simulink model "Lecture_2_Exercises_Simulink"  (R2023b)
settings: Solver=ode3  StartTime=0.0  StopTime=100  FixedStep=0.001  RelTol=1e-3
values from neighbouring files (symbols this model uses):
  A = [ 0 1 ; -g/l*cos(pi/4) -d/(m*l^2) ]    [Lecture_2_Exercises.m]
  a = [m ... (first row only)    [Lecture_2_Exercises.m]
  B = [ 0 ; 1/(m*l^2) ]    [Lecture_2_Exercises.m]
  ustar = m*g*l*sin(xstar(1))    [Lecture_2_Exercises.m]
  xstar = [pi/4 ... (first row only)    [Lecture_2_Exercises.m]
libraries: simulink_extras x4
settings Model: Creator=therk  LastModifiedBy=therk

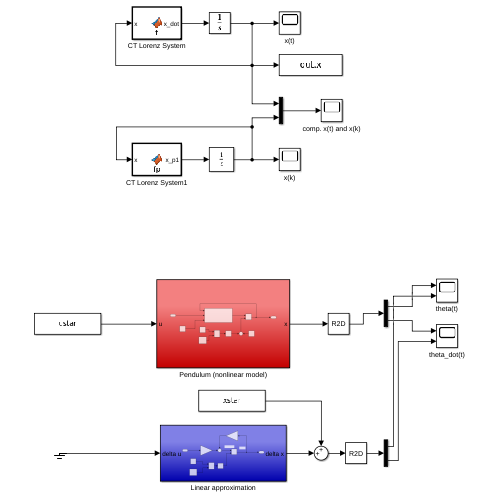
[thumbnail: Simulink's stored preview of the top-level diagram]
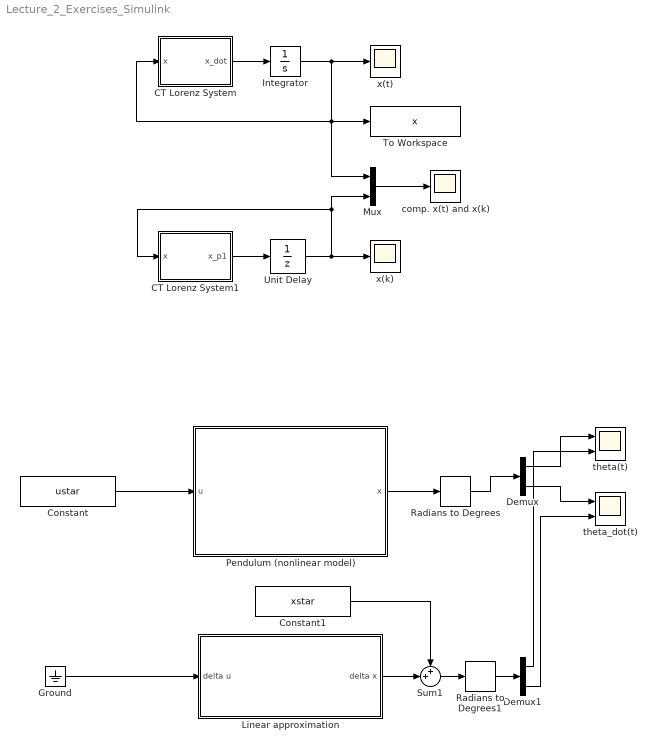
== system Lecture_2_Exercises_Simulink ==
  CT Lorenz System : MATLAB Function  TreatAsAtomicUnit=on
  CT Lorenz System1 : MATLAB Function  TreatAsAtomicUnit=on
  Constant : Constant  Value=ustar
  Constant1 : Constant  Value=xstar  VectorParams1D=off
  Demux : Demux  Outputs=2
  Demux1 : Demux  Outputs=2
  Ground : Ground
  Integrator : Integrator  InitialCondition=[0;1;0]
  Linear approximation : Subsystem
  Mux : Mux  Inputs=2
  Pendulum (nonlinear model) : Subsystem
  Radians to Degrees : simulink_extras/Transformations/Radians to Degrees
  Radians to Degrees1 : simulink_extras/Transformations/Radians to Degrees
  Sum1 : Sum  Inputs=++|
  To Workspace : ToWorkspace  VariableName=x  SampleTime=-1
  Unit Delay : UnitDelay  InitialCondition=[0;1;0]  SampleTime=1e-3  HasFrameUpgradeWarning=on
  comp. x(t) and x(k) : Scope
  theta(t) : Scope  NumInputPorts=2
  theta_dot(t) : Scope  NumInputPorts=2
  x(k) : Scope
  x(t) : Scope
  wires:
  CT Lorenz System/1(x_dot) -> Integrator/1
  Integrator/1 -> x(t)/1, Mux/1, CT Lorenz System/1(x), To Workspace/1
  CT Lorenz System1/1(x_p1) -> Unit Delay/1
  Unit Delay/1 -> Mux/2, CT Lorenz System1/1(x), x(k)/1
  Mux/1 -> comp. x(t) and x(k)/1
  Constant1/1 -> Sum1/1
  Ground/1 -> Linear approximation/1(delta u)
  Linear approximation/1(delta x) -> Sum1/2
  Radians to Degrees/1 -> Demux/1
  Demux1/2 -> theta_dot(t)/2
  Pendulum (nonlinear model)/1(x) -> Radians to Degrees/1
  Radians to Degrees1/1 -> Demux1/1
  Demux/1 -> theta(t)/1
  Sum1/1 -> Radians to Degrees1/1
  Constant/1 -> Pendulum (nonlinear model)/1(u)
  Demux/2 -> theta_dot(t)/1
  Demux1/1 -> theta(t)/2

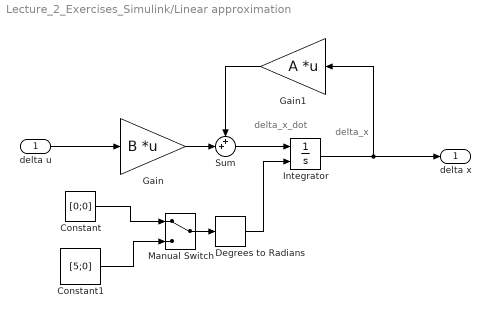
== system Lecture_2_Exercises_Simulink/Linear approximation ==
  note: delta_x_dot
  note: delta_x
  delta u : Inport
  Constant : Constant  Value=[0;0]  VectorParams1D=off
  Constant1 : Constant  Value=[5;0]  VectorParams1D=off
  Degrees to Radians : simulink_extras/Transformations/Degrees to Radians
  Gain : Gain  Gain=B  Multiplication=Matrix(K*u) (u vector)
  Gain1 : Gain  Gain=A  Multiplication=Matrix(K*u) (u vector)
  Integrator : Integrator  InitialConditionSource=external  InitialCondition=[0.5;0]
  Manual Switch : ManualSwitch
  Sum : Sum  Inputs=++|
  delta x : Outport
  wires:
  delta u/1 -> Gain/1
  Sum/1 -> Integrator/1
  Integrator/1 -> Gain1/1, delta x/1
  Gain1/1 -> Sum/1
  Gain/1 -> Sum/2
  Manual Switch/1 -> Degrees to Radians/1
  Constant/1 -> Manual Switch/1
  Constant1/1 -> Manual Switch/2
  Degrees to Radians/1 -> Integrator/2

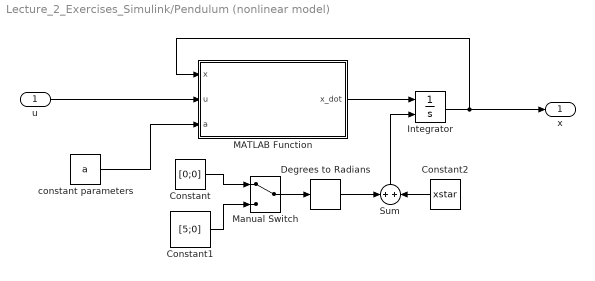
== system Lecture_2_Exercises_Simulink/Pendulum (nonlinear model) ==
  u : Inport
  Constant : Constant  Value=[0;0]  VectorParams1D=off
  Constant1 : Constant  Value=[5;0]  VectorParams1D=off
  Constant2 : Constant  Value=xstar  VectorParams1D=off
  Degrees to Radians : simulink_extras/Transformations/Degrees to Radians
  Integrator : Integrator  InitialConditionSource=external  InitialCondition=xstar
  MATLAB Function : MATLAB Function  TreatAsAtomicUnit=on
  Manual Switch : ManualSwitch
  Sum : Sum
  constant parameters : Constant  Value=a  VectorParams1D=off
  x : Outport
  wires:
  u/1 -> MATLAB Function/2(u)
  MATLAB Function/1(x_dot) -> Integrator/1
  Integrator/1 -> MATLAB Function/1(x), x/1
  constant parameters/1 -> MATLAB Function/3(a)
  Constant/1 -> Manual Switch/1
  Constant1/1 -> Manual Switch/2
  Manual Switch/1 -> Degrees to Radians/1
  Sum/1 -> Integrator/2
  Constant2/1 -> Sum/2
  Degrees to Radians/1 -> Sum/1

== matlab function Lecture_2_Exercises_Simulink/CT Lorenz System ==
  data: x input; x_dot output
function x_dot = f(x) % nonlinear mapping

rho = 28;
sigma = 10;
beta = 8/3;

x_dot = [ sigma*(x(2) - x(1))  ;
          x(1)*(rho-x(3))-x(2) ; 
          x(1)*x(2)-beta*x(3) ];

== matlab function Lecture_2_Exercises_Simulink/Pendulum (nonlinear model)/MATLAB Function ==
  data: x input; u input; x_dot output; a input
function x_dot = f(x,u,a)

% a is the vector of constant parameters
m = a(1);
g = a(2);
l = a(3);
d = a(4);

x_dot = [ x(2) ; 1/(m*l^2)*(-m*g*l*sin(x(1))-d*x(2)+u) ];

== matlab function Lecture_2_Exercises_Simulink/CT Lorenz System1 ==
  data: x input; x_p1 output
function x_p1 = fp(x) % nonlinear mapping f "prime" (discrete-time)
% x_p1 means x(k+1)
rho = 28;
sigma = 10;
beta = 8/3;

Ts = 1e-3; % sampling time

x_p1 = x + Ts*[ sigma*(x(2) - x(1))  ;
                x(1)*(rho-x(3))-x(2) ; 
                x(1)*x(2)-beta*x(3) ];
